simulink model "HevP2ReferenceApplication"  (R2022a)
settings: Solver=ode23tb  StartTime=0  StopTime=2474  RelTol=1e-2  EnableMultiTasking=on
undefined symbols (not defined in the file or in its folder): sigbuilder_block, SOCLast
libraries: simulink x5, autolibshared x2
(part 1 of 2)
settings Model: DataDictionary=HevP2ReferenceApplication.sldd  ModifiedByFormat=The MathWorks, Inc.  SimulationMode=accelerator  PauseTimes=23.46  Creator=The MathWorks, Inc.  LastModifiedBy=The MathWorks, Inc.
settings SolverCC: MaxConsecutiveMinStep=50  SolverJacobianMethodControl=FullPerturbation  ZeroCrossAlgorithm=Adaptive  AlgebraicLoopSolver=TrustRegion  AutoInsertRateTranBlk=on  DecoupledContinuousIntegration=on  MinimalZcImpactIntegration=on  MaxZcPerStep=1
settings DataIOCC: SaveOutput=off  DSMLogging=off  SaveTime=off  ReturnWorkspaceOutputs=off
settings OptimizationCC: EfficientMapNaN2IntZero=off
settings DebuggingCC: UnderspecifiedInitializationDetection=Classic  MergeDetectMultiDrivingBlocksExec=none  MaskedZcDiagnostic=none  IgnoredZcDiagnostic=none  UnconnectedInputMsg=warning  UnconnectedOutputMsg=warning  UnconnectedLineMsg=warning  ModelReferenceExtraNoncontSigs=none  PregeneratedLibrarySubsystemCodeDiagnostic=none  SFMachineParentedDataDiag=warning  ArithmeticOperatorsInVariantConditions=warning
settings HardwareCC: TargetBitPerLong=64  TargetBitPerPointer=64  TargetBitPerSizeT=64  TargetBitPerPtrDiffT=64  TargetLongLongMode=on  TargetIntDivRoundTo=Zero  TargetEndianess=LittleEndian  TargetWordSize=64  TargetHWDeviceType=MATLAB Host  ProdEqTarget=off
settings ModelReferenceCC: UpdateModelReferenceTargets=IfOutOfDate  ModelReferenceMinAlgLoopOccurrences=on  PropagateSignalLabelsOutOfModel=off
settings SFSimCC: SimUseLocalCustomCode=off
settings RTWCC: RTWUseLocalCustomCode=off  DLArmComputeVersion=19.05
settings CodeAppCC: MaxIdLength=128
settings GRTTargetCC: TargetLangStandard=C89/C90 (ANSI)  CombineOutputUpdateFcns=off  GRTInterface=on
settings ConfigComp: CovMetricSettings=dsw  CovSaveCumulativeToWorkspaceVar=on  CovSaveSingleToWorkspaceVar=on  CovExternalEMLEnable=off

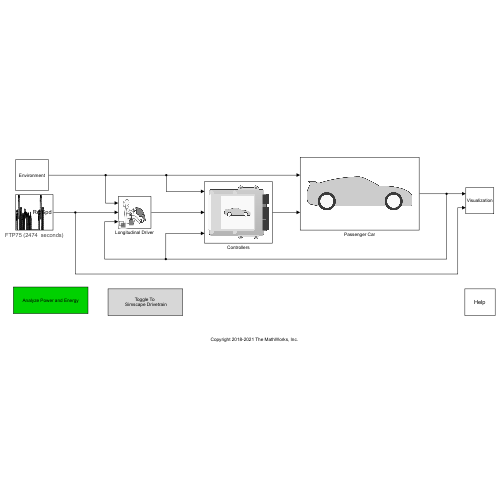
[thumbnail: Simulink's stored preview of the top-level diagram]
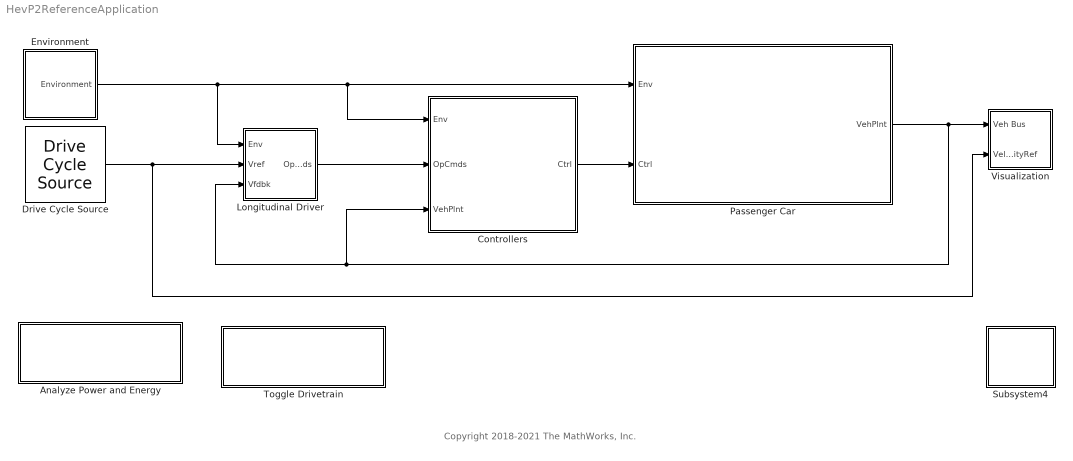
== system HevP2ReferenceApplication ==
  note: Copyright 2018-2021 The MathWorks, Inc.
  Analyze Power and Energy : Subsystem
      settings: OpenFcn=edit GenerateEnergyReport
      mask Display: disp(getString(message('autoblks:autoblkVehMask:powAndEne')))
  Controllers : Subsystem
      mask Display: image('SystemControllers.png', 'center')
  Drive Cycle Source : autolibshared/Drive Cycle Source  cycleVar=FTP75  fileVar=L:\Bauto\matlab\test\toolbox\shared\autoblks\scenario\adac.txt  tfinal="2474  seconds"  cycleRepeat=off  outAccPort=off  outGearPort=off  gearList=No gear data  t_wot1=1  xdot_woto=0  xdot_wot1=26.8  t_wot2=30  xdot_wot2=0  t_wotend=40  srcUnit=m/s  outUnit=m/s  srcAccUnit=m/s/s  outAccUnit=m/s^2  dt=0  aMode=1  faultOption=off  velBnd=2  velBndUnit=mph  inUnit=m/s  timeBnd=1  failOption=off  stopSim=off  maxFaultCnt=10  maxFaultTime=2  maxTotFaultTime=15  traceOption=off  dtTrace=1  traceWindow=10  lastDCname=FTP75  lastOutUnit=mph  lastDT=0  lastTB=1  lastSB=2  forceCalcBound=off
      settings: SourceProductBaseCode=PW,DR,MT,VE
  Environment : Subsystem
      mask Display: disp(getString(message('autoblks:autoblkVehMask:environ')))
  Longitudinal Driver : Subsystem  Variant=on  VariantControlMode=label  VariantControl=Variant1  LabelModeActiveChoice=0
      mask Display:
      | if strcmp('1',get_param(gcb,'ActiveVariant'))
      |     disp('Open Loop')
      | else
      |     image('LongitudinalDriver.png','center');
      | end
  Passenger Car : Subsystem
      mask Display: image('PassengerVehicle.png', 'center')
  Subsystem4 : Subsystem
      settings: OpenFcn=helpview([docroot,'/toolbox/autoblks/helptargets.map'], 'p2_hybrid_refapp')
      mask Display: disp(getString(message('autoblks:autoblkVehMask:help')))
  Toggle Drivetrain : Subsystem  mask(Drivetrain Model Selection){drivetrainMode=Powertrain Blockset}
      mask help: autoblks:autoblkHEVPx:ToggleDrivetrainSimscapeDesc
      settings: OpenFcn=open_system(gcb,'Mask')
      mask Help: eval('autosharedhelp(''p2_hybrid_refapp'')');
      mask TypeOptions drivetrainMode: Powertrain Blockset | Simscape
      mask Callback drivetrainMode:
      | if(strcmp(get_param(bdroot,'simulationstatus'),'stopped')) % only execute if simulation is stopped
      |     switch get_param(gcb,'drivetrainMode')
      |         case "Powertrain Blockset"
      |             set_param(bdroot,'Solver','ode23tb')
      |             set_param([bdroot '/Passenger Car/Drivetrain'], 'OverrideUsingVariant', 'Powertrain Blockset');
      |         case "Simscape"
      |             set_param(bdroot,'Solver','ode23t')
      |             set_param([bdroot '/Passenger Car/Drivetrain'], 'OverrideUsingVariant', 'Simscape');
      |         otherwise
      |             set_param(bdroot,'Solver','ode23tb')
      |             set_param([bdroot '/Passenger Car/Drivetrain'], 'OverrideUsingVariant', 'PTBS');
      |     end
      | end
      mask DialogControl ParameterGroupVar Prompt: Model Type
      mask Display:
      | if strcmp(get_param([bdroot(gcb) '/Passenger Car/Drivetrain'],'LabelModeActiveChoice'),'Powertrain Blockset')
      |    disp('Toggle To \n Simscape Drivetrain');
      | else
      |    disp('Toggle To \n Powertrain Blockset Drivetrain');
      | end
  Visualization : Subsystem
      mask Display: disp(getString(message('autoblks:autoblkVehMask:visual')))
  wires:
  Longitudinal Driver/1(" OpCmds") -> Controllers/2(OpCmds)
  Drive Cycle Source/1 -> Visualization/2(VelocityRef), Longitudinal Driver/2("Vref ")
  Environment/1(Environment) -> Passenger Car/1(Env), Controllers/1(Env), Longitudinal Driver/1(Env)
  Controllers/1(Ctrl) -> Passenger Car/2(Ctrl)
  Passenger Car/1(VehPlnt) -> Longitudinal Driver/3("Vfdbk "), Controllers/3(VehPlnt), Visualization/1(Veh Bus)

== system HevP2ReferenceApplication/Analyze Power and Energy ==

== system HevP2ReferenceApplication/Controllers ==
  Env : Inport
  OpCmds : Inport  Port=2
  VehPlnt : Inport  Port=3
  Bus Creator : BusCreator  Inputs=2
  PCM Input : Subsystem
  PCM Output : Subsystem
  Powertrain Control Module (PCM) : Subsystem
  Ctrl : Outport  VectorParamsAs1DForOutWhenUnconnected=off
  wires:
  Bus Creator/1 -> Ctrl/1
  [EngCtrl] -> Bus Creator/1
  [PtCtrl] -> Bus Creator/2
  Env/1 -> [Environment]
  VehPlnt/1 -> [VehPlnt]
  OpCmds/1 -> [OpCmds]
  PCM Input/27(BattSoc) -> Powertrain Control Module (PCM)/27(BattSoc)
  PCM Input/22(Ect) -> Powertrain Control Module (PCM)/22(Ect)
  PCM Input/23(EgrDeltaPrs) -> Powertrain Control Module (PCM)/23(EgrVlvDeltaPrs)
  PCM Input/5(ThrPosPct) -> Powertrain Control Module (PCM)/5(ThrPosPct)
  Powertrain Control Module (PCM)/7(ExhCamPhaseCmd) -> PCM Output/7(ExhCamPhaseCmd)
  PCM Input/32(EngTrqOut) -> Powertrain Control Module (PCM)/32(EngTrqOut)
  PCM Input/24(EgrInTemp) -> Powertrain Control Module (PCM)/24(EgrVlvInTemp)
  PCM Input/25(VehSpdFdbk) -> Powertrain Control Module (PCM)/25(VehSpdFdbk)
  PCM Input/12(IntkVlvLift) -> Powertrain Control Module (PCM)/12(IntkVlvLift)
  PCM Input/11(VarCompRatioPos) -> Powertrain Control Module (PCM)/11(VarCompRatioPos)
  PCM Input/26(EngSpdFdbk) -> Powertrain Control Module (PCM)/26(EngSpdFdbk)
  PCM Input/15(IntkSwirlVlvPos) -> Powertrain Control Module (PCM)/15(IntkSwirlVlvPos)
  Powertrain Control Module (PCM)/5(SpdAdv) -> PCM Output/5(SpkAdv)
  Powertrain Control Module (PCM)/13(ClsdLpFuelMult) -> PCM Output/13(ClsdLpFuelMult)
  PCM Input/28(BattPwr) -> Powertrain Control Module (PCM)/28(BattPwr)
  PCM Input/16(TurboSpd) -> Powertrain Control Module (PCM)/16(TurboSpd)
  PCM Input/10(EgrVlvAreaPct) -> Powertrain Control Module (PCM)/10(EgrVlvAreaPct)
  PCM Input/9(TurboRackPos) -> Powertrain Control Module (PCM)/9(TurboRackPos)
  PCM Input/14(Afr) -> Powertrain Control Module (PCM)/14(Afr)
  PCM Input/17(AmbPrs) -> Powertrain Control Module (PCM)/17(AmbPrs)
  PCM Input/13(VarIntkRunLen) -> Powertrain Control Module (PCM)/13(VarIntkRunLen)
  PCM Input/21(Iat) -> Powertrain Control Module (PCM)/21(Iat)
  Powertrain Control Module (PCM)/15(TrqCmdISC) -> PCM Output/15(TrqCmdISC)
  PCM Input/18(AccelPdl) -> Powertrain Control Module (PCM)/18(AccelPdl)
  Powertrain Control Module (PCM)/4(FuelMainSoi) -> PCM Output/4(FuelMainSoi)
  [Environment] -> PCM Input/2(Env)
  PCM Input/6(WgAreaPct) -> Powertrain Control Module (PCM)/6(WgAreaPct)
  Powertrain Control Module (PCM)/12(VarIntkRunLenCmd) -> PCM Output/12(VarIntkRunLenCmd)
  PCM Input/19(DecelPdl) -> Powertrain Control Module (PCM)/19(DecelPdl)
  PCM Input/1(TrqCmd) -> Powertrain Control Module (PCM)/1(TrqCmd)
  PCM Input/4(Mat) -> Powertrain Control Module (PCM)/4(Mat)
  Powertrain Control Module (PCM)/11(IntkVlvLiftCmd) -> PCM Output/11(IntkVlvLiftCmd)
  Powertrain Control Module (PCM)/18(EngTrqCmd) -> PCM Output/18(EngTrqCmd)
  PCM Input/3(Map) -> Powertrain Control Module (PCM)/3(Map)
  Powertrain Control Module (PCM)/21(BrkCmd) -> PCM Output/21(BrkCmd)
  PCM Input/20(IgnSwtch) -> Powertrain Control Module (PCM)/20(IgnSwtch)
  Powertrain Control Module (PCM)/16(LoadCmd) -> PCM Output/16(LoadCmd)
  PCM Input/7(IntkCamPhase) -> Powertrain Control Module (PCM)/7(IntkCamPhase)
  [PtCtrl] -> PCM Input/1(PtCtrl)
  Powertrain Control Module (PCM)/6(IntkCamPhaseCmd) -> PCM Output/6(IntkCamPhaseCmd)
  PCM Output/2(PtCtrl) -> [PtCtrl]
  Powertrain Control Module (PCM)/19(StartCmd) -> PCM Output/19(StartCmd)
  PCM Input/2(EngSpd) -> Powertrain Control Module (PCM)/2(EngSpd)
  Powertrain Control Module (PCM)/10(VarCompRatioPosCmd) -> PCM Output/10(VarCompRatioPosCmd)
  Powertrain Control Module (PCM)/17(EstIntkPortFlw) -> PCM Output/17(EstIntkPortFlw)
  [VehPlnt] -> PCM Input/3(VehPlnt)
  Powertrain Control Module (PCM)/9(EgrVlvAreaPctCmd) -> PCM Output/9(EgrVlvAreaPctCmd)
  Powertrain Control Module (PCM)/1(ThrPosPctCmd) -> PCM Output/1(ThrPosPctCmd)
  Powertrain Control Module (PCM)/2(WgAreaPctCmd) -> PCM Output/2(WgAreaPctCmd)
  [OpCmds] -> PCM Input/4(OpCmds)
  PCM Input/8(ExhCamPhase) -> Powertrain Control Module (PCM)/8(ExhCamPhase)
  Powertrain Control Module (PCM)/3(InjPw) -> PCM Output/3(InjPw)
  Powertrain Control Module (PCM)/14(IntkSwirlVlvPosCmd) -> PCM Output/14(IntkSwirlVlvPosCmd)
  PCM Input/29(MotSpd) -> Powertrain Control Module (PCM)/29(MotSpd)
  Powertrain Control Module (PCM)/8(TurboRackPosCmd) -> PCM Output/8(TurboRackPosCmd)
  PCM Output/1(EngCtrl) -> [EngCtrl]
  PCM Input/30(Cltch1State) -> Powertrain Control Module (PCM)/30(Cltch1State)
  PCM Input/31(Cltch2State) -> Powertrain Control Module (PCM)/31(Cltch2State)
  Powertrain Control Module (PCM)/22(GearCmd) -> PCM Output/22(GearCmd)
  Powertrain Control Module (PCM)/23(Cltch1Cmd) -> PCM Output/23(Cltch1Cmd)
  PCM Input/33(Chrg) -> Powertrain Control Module (PCM)/33(Chrg)
  Powertrain Control Module (PCM)/20(MotTrqCmd) -> PCM Output/20(MotTrqCmd)
  PCM Input/34(BattV) -> Powertrain Control Module (PCM)/34(BattV)
  PCM Input/35(TransGear) -> Powertrain Control Module (PCM)/35(TransGear)

== system HevP2ReferenceApplication/Environment ==
  Bus Creator : BusCreator  Inputs=4
  Bus Creator3 : BusCreator  Inputs=3
  Bus Creator4 : BusCreator  Inputs=2
  Bus Creator5 : BusCreator  Inputs=2
  Constant2 : Constant  Value=0
  Constant3 : Constant  Value=0
  Constant6 : Constant  Value=300
  Constant7 : Constant  Value=101325
  Ground{,1..3} (4 alike) : Ground
  Environment : Outport  VectorParamsAs1DForOutWhenUnconnected=off
  wires:
  Ground2/1 -> Bus Creator5/1  "lam_mu_x"
  Ground3/1 -> Bus Creator5/2  "lam_mu_y"
  Bus Creator5/1 -> Bus Creator4/2  "Ground_mu"
  Bus Creator4/1 -> Bus Creator/3  "Ground"
  Bus Creator3/1 -> Bus Creator/4  "Wind"
  Constant3/1 -> Bus Creator3/1  "wind_x"
  Ground/1 -> Bus Creator3/2  "wind_y"
  Ground1/1 -> Bus Creator3/3  "wind_z"
  Constant6/1 -> Bus Creator/1  "Temp"
  Constant2/1 -> Bus Creator4/1  "Grade"
  Bus Creator/1 -> Environment/1  "Environment"
  Constant7/1 -> Bus Creator/2  "Baro"

== system HevP2ReferenceApplication/Longitudinal Driver ==
  note: To switch variants, right-click on this subsystem (from one level above) and chose:
      | Variant, Active choice, <your selection>
  Env : Inport
  "Vref " : Inport  Port=2
  "Vfdbk " : Inport  Port=3
  Longitudinal Driver : Subsystem  VariantControl=0
      mask Display: image('LongitudinalDriver.png', 'center')
  Open Loop : Subsystem  VariantControl=1
      mask Display: disp('Open Loop')
  " OpCmds" : Outport  VectorParamsAs1DForOutWhenUnconnected=off

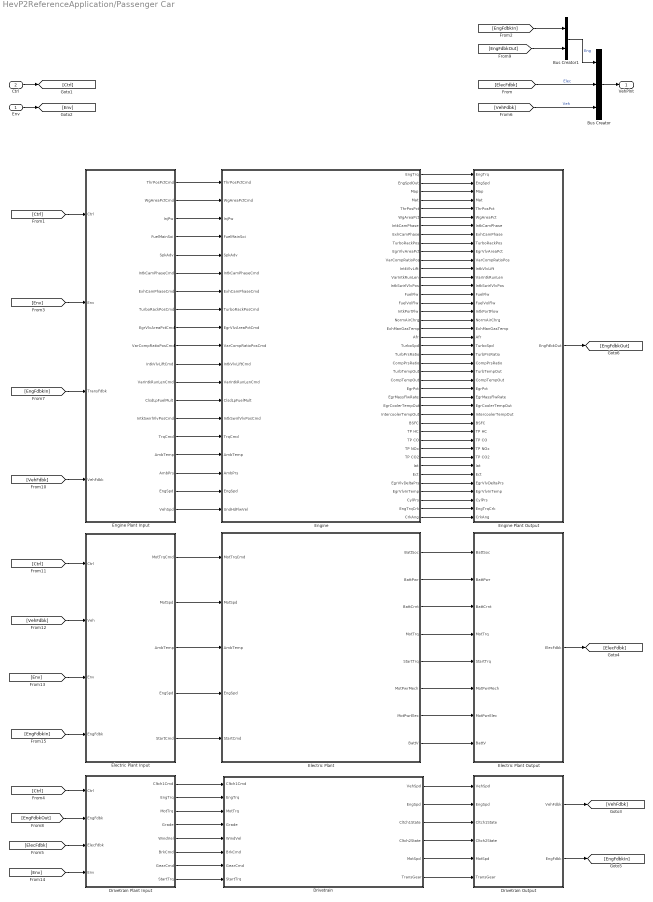
== system HevP2ReferenceApplication/Passenger Car ==
  Env : Inport
  Ctrl : Inport  Port=2
  Bus Creator : BusCreator  Inputs=3
  Bus Creator1 : BusCreator  Inputs=2
  Drivetrain : Subsystem  Variant=on  VariantControlMode=label  LabelModeActiveChoice=Powertrain Blockset
  Drivetrain Output : Subsystem
  Drivetrain Plant Input : Subsystem
  Electric Plant : Subsystem
  Electric Plant Input : Subsystem
  Electric Plant Output : Subsystem
  Engine : Subsystem  Variant=on  VariantControlMode=label  LabelModeActiveChoice=SiMappedEngine
  Engine Plant Input : Subsystem
  Engine Plant Output : Subsystem
  VehPlnt : Outport  VectorParamsAs1DForOutWhenUnconnected=off
  wires:
  [Ctrl] -> Drivetrain Plant Input/1(Ctrl)
  [EngFdbkOut] -> Drivetrain Plant Input/2(EngFdbk)
  Drivetrain/1(VehSpd) -> Drivetrain Output/1(VehSpd)
  Electric Plant Output/1(ElecFdbk) -> [ElecFdbk]
  [Ctrl] -> Electric Plant Input/1(Ctrl)
  [ElecFdbk] -> Drivetrain Plant Input/3(ElecFdbk)
  Drivetrain Plant Input/3(MotTrq) -> Drivetrain/3(MotTrq)
  Drivetrain Plant Input/1(Cltch1Cmd) -> Drivetrain/1(Cltch1Cmd)
  Drivetrain Plant Input/2(EngTrq) -> Drivetrain/2(EngTrq)
  [VehFdbk] -> Electric Plant Input/2(Veh)
  Electric Plant Input/1(MotTrqCmd) -> Electric Plant/1(MotTrqCmd)
  Electric Plant Input/2(MotSpd) -> Electric Plant/2(MotSpd)
  Electric Plant/1(BattSoc) -> Electric Plant Output/1(BattSoc)
  Electric Plant/2(BattPwr) -> Electric Plant Output/2(BattPwr)
  Electric Plant/3(BattCrnt) -> Electric Plant Output/3(BattCrnt)
  Electric Plant/4(MotTrq) -> Electric Plant Output/4(MotTrq)
  [Env] -> Electric Plant Input/3(Env)
  Electric Plant Input/3(AmbTemp) -> Electric Plant/3(AmbTemp)
  [Env] -> Drivetrain Plant Input/4(Env)
  Drivetrain Plant Input/4(Grade) -> Drivetrain/4(Grade)
  Drivetrain Plant Input/5(WindVel) -> Drivetrain/5(WindVel)
  [EngFdbkIn] -> Electric Plant Input/4(EngFdbk)
  Electric Plant Input/4(EngSpd) -> Electric Plant/4(EngSpd)
  Electric Plant/5(StartTrq) -> Electric Plant Output/5(StartTrq)
  Electric Plant Input/5(StartCmd) -> Electric Plant/5(StartCmd)
  Engine Plant Input/17(AmbPrs) -> Engine/17(AmbPrs)
  [EngFdbkIn] -> Bus Creator1/1
  Engine Plant Input/6(IntkCamPhaseCmd) -> Engine/6(IntkCamPhaseCmd)
  Engine Plant Input/12(VarIntkRunLenCmd) -> Engine/12(VarIntkRunLenCmd)
  [EngFdbkIn] -> Engine Plant Input/3(TransFdbk)
  Engine Plant Input/16(AmbTemp) -> Engine/16(AmbTemp)
  Bus Creator/1 -> VehPlnt/1
  Engine Plant Input/14(IntkSwirlVlvPosCmd) -> Engine/14(IntkSwirlVlvPosCmd)
  [ElecFdbk] -> Bus Creator/2  "Elec"
  Engine Plant Input/5(SpkAdv) -> Engine/5(SpkAdv)
  Engine Plant Output/1(EngFdbkOut) -> [EngFdbkOut]
  Env/1 -> [Env]
  [EngFdbkOut] -> Bus Creator1/2
  Engine Plant Input/7(ExhCamPhaseCmd) -> Engine/7(ExhCamPhaseCmd)
  Engine Plant Input/1(ThrPosPctCmd) -> Engine/1(ThrPosPctCmd)
  Engine Plant Input/19(VehSpd) -> Engine/19(UndHdFlwVel)
  Engine Plant Input/9(EgrVlvAreaPctCmd) -> Engine/9(EgrVlvAreaPctCmd)
  [Env] -> Engine Plant Input/2(Env)
  Engine Plant Input/3(InjPw) -> Engine/3(InjPw)
  Engine Plant Input/11(IntkVlvLiftCmd) -> Engine/11(IntkVlvLiftCmd)
  [VehFdbk] -> Engine Plant Input/4(VehFdbk)
  Engine Plant Input/4(FuelMainSoi) -> Engine/4(FuelMainSoi)
  Engine Plant Input/18(EngSpd) -> Engine/18(EngSpd)
  Engine Plant Input/8(TurboRackPosCmd) -> Engine/8(TurboRackPosCmd)
  Engine Plant Input/2(WgAreaPctCmd) -> Engine/2(WgAreaPctCmd)
  [Ctrl] -> Engine Plant Input/1(Ctrl)
  Engine Plant Input/13(ClsdLpFuelMult) -> Engine/13(ClsdLpFuelMult)
  Engine Plant Input/10(VarCompRatioPosCmd) -> Engine/10(VarCompRatioPosCmd)
  Bus Creator1/1 -> Bus Creator/1  "Eng"
  Ctrl/1 -> [Ctrl]
  Engine Plant Input/15(TrqCmd) -> Engine/15(TrqCmd)
  [VehFdbk] -> Bus Creator/3  "Veh"
  Electric Plant/6(MotPwrMech) -> Electric Plant Output/6(MotPwrMech)
  Electric Plant/7(MotPwrElec) -> Electric Plant Output/7(MotPwrElec)
  Electric Plant/8(BattV) -> Electric Plant Output/8(BattV)
  Engine/1(EngTrq) -> Engine Plant Output/1(EngTrq)
  Engine/2(EngSpdOut) -> Engine Plant Output/2(EngSpd)
  Engine/3(Map) -> Engine Plant Output/3(Map)
  Engine/4(Mat) -> Engine Plant Output/4(Mat)
  Engine/5(ThrPosPct) -> Engine Plant Output/5(ThrPosPct)
  Engine/6(WgAreaPct) -> Engine Plant Output/6(WgAreaPct)
  Engine/7(IntkCamPhase) -> Engine Plant Output/7(IntkCamPhase)
  Engine/8(ExhCamPhase) -> Engine Plant Output/8(ExhCamPhase)
  Engine/9(TurboRackPos) -> Engine Plant Output/9(TurboRackPos)
  Engine/10(EgrVlvAreaPct) -> Engine Plant Output/10(EgrVlvAreaPct)
  Engine/11(VarCompRatioPos) -> Engine Plant Output/11(VarCompRatioPos)
  Engine/12(IntkVlvLift) -> Engine Plant Output/12(IntkVlvLift)
  Engine/13(VarIntkRunLen) -> Engine Plant Output/13(VarIntkRunLen)
  Engine/14(IntkSwirlVlvPos) -> Engine Plant Output/14(IntkSwirlVlvPos)
  Engine/15(FuelFlw) -> Engine Plant Output/15(FuelFlw)
  Engine/16(FuelVolFlw) -> Engine Plant Output/16(FuelVolFlw)
  Engine/17(IntkPortFlw) -> Engine Plant Output/17(IntkPortFlow)
  Engine/18(NormAirChrg) -> Engine Plant Output/18(NormAirChrg)
  Engine/19(ExhManGasTemp) -> Engine Plant Output/19(ExhManGasTemp)
  Engine/20(Afr) -> Engine Plant Output/20(Afr)
  Engine/21(TurboSpd) -> Engine Plant Output/21(TurboSpd)
  Engine/22(TurbPrsRatio) -> Engine Plant Output/22(TurbPrsRatio)
  Engine/23(CompPrsRatio) -> Engine Plant Output/23(CompPrsRatio)
  Engine/24(TurbTempOut) -> Engine Plant Output/24(TurbTempOut)
  Engine/25(CompTempOut) -> Engine Plant Output/25(CompTempOut)
  Engine/26(EgrPct) -> Engine Plant Output/26(EgrPct)
  Engine/27(EgrMassFlwRate) -> Engine Plant Output/27(EgrMassFlwRate)
  Engine/28(EgrCoolerTempOut) -> Engine Plant Output/28(EgrCoolerTempOut)
  Engine/29(IntercoolerTempOut) -> Engine Plant Output/29(IntercoolerTempOut)
  Engine/30(BSFC) -> Engine Plant Output/30(BSFC)
  Engine/31(TP HC) -> Engine Plant Output/31(TP HC)
  Engine/32(TP CO) -> Engine Plant Output/32(TP CO)
  Engine/33(TP NOx) -> Engine Plant Output/33(TP NOx)
  Engine/34(TP CO2) -> Engine Plant Output/34(TP CO2)
  Engine/35(Iat) -> Engine Plant Output/35(Iat)
  Engine/36(Ect) -> Engine Plant Output/36(Ect)
  Engine/37(EgrVlvDeltaPrs) -> Engine Plant Output/37(EgrVlvDeltaPrs)
  Engine/38(EgrVlvInTemp) -> Engine Plant Output/38(EgrVlvInTemp)
  Engine/39(CylPrs) -> Engine Plant Output/39(CylPrs)
  Engine/40(EngTrqCrk) -> Engine Plant Output/40(EngTrqCrk)
  Engine/41(CrkAng) -> Engine Plant Output/41(CrkAng)
  Drivetrain/4(Cltch2State) -> Drivetrain Output/4(Cltch2State)
  Drivetrain/3(Cltch1State) -> Drivetrain Output/3(Cltch1State)
  Drivetrain Output/2(EngFdbk) -> [EngFdbkIn]
  Drivetrain Output/1(VehFdbk) -> [VehFdbk]
  Drivetrain/6(TransGear) -> Drivetrain Output/6(TransGear)
  Drivetrain/2(EngSpd) -> Drivetrain Output/2("EngSpd ")
  Drivetrain/5(MotSpd) -> Drivetrain Output/5(MotSpd)
  Drivetrain Plant Input/7(GearCmd) -> Drivetrain/7(GearCmd)
  Drivetrain Plant Input/8(StartTrq) -> Drivetrain/8(StartTrq)
  Drivetrain Plant Input/6(BrkCmd) -> Drivetrain/6(BrkCmd)

== system HevP2ReferenceApplication/Subsystem4 ==

== system HevP2ReferenceApplication/Toggle Drivetrain ==

== system HevP2ReferenceApplication/Visualization ==
  Veh Bus : Inport
  VelocityRef : Inport  Port=2
  Bus Selector1 : BusSelector  OutputSignals=Veh.xdot,Eng.EngFdbkOut.EngSpd,Veh.MotSpd,Eng.EngFdbkOut.EngTrq,Elec.MotTrq,Elec.BattCrnt,Elec.BattSoc,Eng.EngFdbkOut.Afr,Eng.EngFdbkOut.FuelVolFlw,Elec.BattPwr,Eng.EngFdbkOut.TP HC,Eng.EngFdbkOut.TP CO,Eng.EngFdbkOut.TP NOx,Eng.EngFdbkOut.TP CO2
  Emission Calculations : Subsystem
  Mux : Mux  Inputs=2
  Mux1 : Mux  Inputs=2
  Mux2 : Mux  Inputs=2
  Performance Calculations : Subsystem
  Performance and FE Scope : Scope  NumInputPorts=6
  Rate Transition{1..2,4..5,7..8,10} (7 alike) : RateTransition  Deterministic=off
  TP Emissions Scope : Scope  NumInputPorts=4
  Terminator : Terminator
  Terminator1 : Terminator
  m/s to mph : Gain  Gain=2.23694
  rad/s to rpm : Gain  Gain=30/pi
  wires:
  Veh Bus/1 -> Bus Selector1/1
  Bus Selector1/1 -> Performance Calculations/1(VehSpd), Mux/2  "<xdot>"
  Bus Selector1/2 -> Rate Transition2/1  "<EngSpd>"
  Mux/1 -> m/s to mph/1
  Bus Selector1/9 -> Performance Calculations/2(FuelVolFlow)  "<FuelVolFlw>"
  Performance Calculations/1(US MPG) -> Performance and FE Scope/6  "US Fuel Economy MPGe"
  Performance Calculations/2(L/100Km) -> Terminator/1
  Bus Selector1/8 -> Terminator1/1  "<Afr>"
  m/s to mph/1 -> Rate Transition4/1
  Bus Selector1/7 -> Rate Transition1/1  "<BattSoc>"
  Bus Selector1/11 -> Emission Calculations/2(TP HC Mass Flow)  "<TP HC>"
  Bus Selector1/12 -> Emission Calculations/3(TP CO Mass Flow)  "<TP CO>"
  Bus Selector1/13 -> Emission Calculations/4(TP NOx Mass Flow)  "<TP NOx>"
  Emission Calculations/1(TP HC Mass) -> TP Emissions Scope/1
  Emission Calculations/2(TP CO Mass) -> TP Emissions Scope/2
  Emission Calculations/3(TP NOx Mass) -> TP Emissions Scope/3
  Bus Selector1/14 -> Emission Calculations/5(TP CO2 Mass Flow)  "<TP CO2>"
  Emission Calculations/4(TP CO2 Mass) -> TP Emissions Scope/4
  VelocityRef/1 -> Emission Calculations/1(VehSpd), Mux/1
  Rate Transition1/1 -> Performance and FE Scope/5  "Battery SOC"
  Mux1/1 -> Performance and FE Scope/2  "EngSpd, MotSpd (RPM)"
  Rate Transition4/1 -> Performance and FE Scope/1  "Trace Velocity, Target, Actual (mph)"
  Bus Selector1/10 -> Performance Calculations/3(BattPwr)  "<BattPwr>"
  Bus Selector1/3 -> rad/s to rpm/1  "<MotSpd>"
  Rate Transition2/1 -> Mux1/1
  Rate Transition5/1 -> Mux1/2
  Rate Transition8/1 -> Mux2/2
  Rate Transition7/1 -> Mux2/1
  Mux2/1 -> Performance and FE Scope/3  "EngTrq, MotTrq (Nm)"
  Bus Selector1/4 -> Rate Transition7/1  "<EngTrq>"
  Bus Selector1/5 -> Rate Transition8/1  "<MotTrq>"
  Bus Selector1/6 -> Rate Transition10/1  "<BattCrnt>"
  Rate Transition10/1 -> Performance and FE Scope/4  "Battery Current (A)"
  rad/s to rpm/1 -> Rate Transition5/1

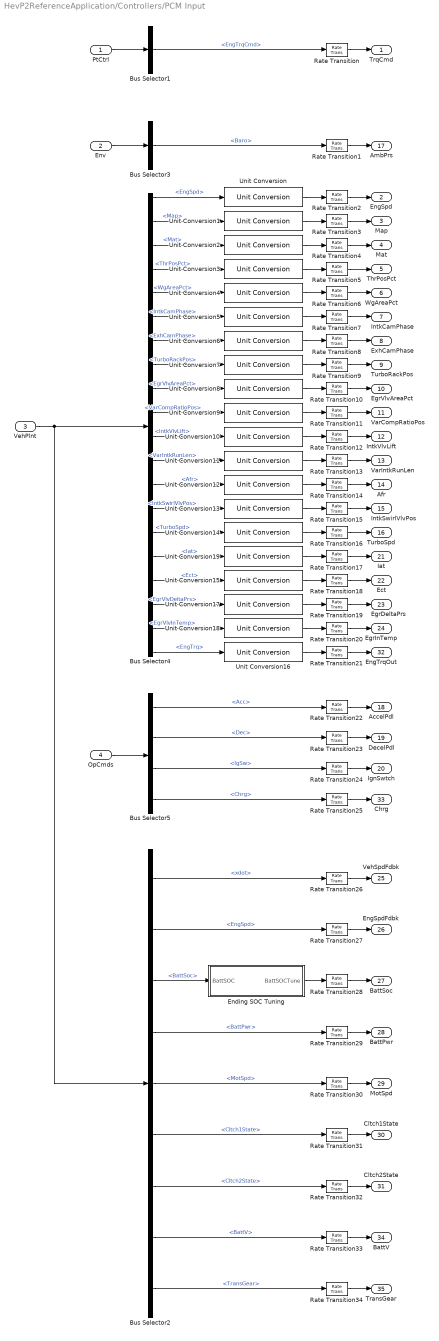
== system HevP2ReferenceApplication/Controllers/PCM Input ==
  PtCtrl : Inport
  Env : Inport  Port=2
  VehPlnt : Inport  Port=3
  OpCmds : Inport  Port=4
  Bus Selector1 : BusSelector  OutputSignals=EngTrqCmd
  Bus Selector2 : BusSelector  OutputSignals=Veh.xdot,Eng.EngFdbk.EngSpd,Elec.BattSoc,Elec.BattPwr,Veh.MotSpd,Veh.Cltch1State,Veh.Cltch2State,Elec.BattV,Veh.TransGear
  Bus Selector3 : BusSelector  OutputSignals=Baro
  Bus Selector4 : BusSelector  OutputSignals=Eng.EngFdbkOut.EngSpd,Eng.EngFdbkOut.Map,Eng.EngFdbkOut.Mat,Eng.EngFdbkOut.ThrPosPct,Eng.EngFdbkOut.WgAreaPct,Eng.EngFdbkOut.IntkCamPhase,Eng.EngFdbkOut.ExhCamPhase,Eng.EngFdbkOut.TurboRackPos,Eng.EngFdbkOut.EgrVlvAreaPct,Eng.EngFdbkOut.VarCompRatioPos,Eng.EngFdbkOut.IntkVlvLift,Eng.EngFdbkOut.VarIntkRunLen,Eng.EngFdbkOut.Afr,Eng.EngFdbkOut.IntkSwirlVlvPos,Eng.EngFdbkOut.TurboSpd,Eng.EngFdbkOut.Iat,Eng.EngFdbkOut.Ect,Eng.EngFdbkOut.EgrVlvDeltaPrs,Eng.EngFdbkOut.EgrVlvInTemp,Eng.EngFdbkOut.EngTrq
  Bus Selector5 : BusSelector  OutputSignals=Acc,Dec,IgSw,Chrg
  Ending SOC Tuning : Subsystem  Variant=on  VariantControlMode=label  LabelModeActiveChoice=0
  Rate Transition{,1..34} (35 alike) : RateTransition
  Unit Conversion{,1..19} (20 alike) : UnitConversion
  TrqCmd : Outport  VectorParamsAs1DForOutWhenUnconnected=off
  EngSpd : Outport  Port=2  VectorParamsAs1DForOutWhenUnconnected=off
  Map : Outport  Port=3  VectorParamsAs1DForOutWhenUnconnected=off
  Mat : Outport  Port=4  VectorParamsAs1DForOutWhenUnconnected=off
  ThrPosPct : Outport  Port=5  VectorParamsAs1DForOutWhenUnconnected=off
  WgAreaPct : Outport  Port=6  VectorParamsAs1DForOutWhenUnconnected=off
  IntkCamPhase : Outport  Port=7  VectorParamsAs1DForOutWhenUnconnected=off
  ExhCamPhase : Outport  Port=8  VectorParamsAs1DForOutWhenUnconnected=off
  TurboRackPos : Outport  Port=9  VectorParamsAs1DForOutWhenUnconnected=off
  EgrVlvAreaPct : Outport  Port=10  VectorParamsAs1DForOutWhenUnconnected=off
  VarCompRatioPos : Outport  Port=11  VectorParamsAs1DForOutWhenUnconnected=off
  IntkVlvLift : Outport  Port=12  VectorParamsAs1DForOutWhenUnconnected=off
  VarIntkRunLen : Outport  Port=13  VectorParamsAs1DForOutWhenUnconnected=off
  Afr : Outport  Port=14  VectorParamsAs1DForOutWhenUnconnected=off
  IntkSwirlVlvPos : Outport  Port=15  VectorParamsAs1DForOutWhenUnconnected=off
  TurboSpd : Outport  Port=16  VectorParamsAs1DForOutWhenUnconnected=off
  AmbPrs : Outport  Port=17  VectorParamsAs1DForOutWhenUnconnected=off
  AccelPdl : Outport  Port=18  VectorParamsAs1DForOutWhenUnconnected=off
  DecelPdl : Outport  Port=19  VectorParamsAs1DForOutWhenUnconnected=off
  IgnSwtch : Outport  Port=20  VectorParamsAs1DForOutWhenUnconnected=off
  Iat : Outport  Port=21  VectorParamsAs1DForOutWhenUnconnected=off
  Ect : Outport  Port=22  VectorParamsAs1DForOutWhenUnconnected=off
  EgrDeltaPrs : Outport  Port=23  VectorParamsAs1DForOutWhenUnconnected=off
  EgrInTemp : Outport  Port=24  VectorParamsAs1DForOutWhenUnconnected=off
  VehSpdFdbk : Outport  Port=25  VectorParamsAs1DForOutWhenUnconnected=off
  EngSpdFdbk : Outport  Port=26  VectorParamsAs1DForOutWhenUnconnected=off
  BattSoc : Outport  Port=27  VectorParamsAs1DForOutWhenUnconnected=off
  BattPwr : Outport  Port=28  VectorParamsAs1DForOutWhenUnconnected=off
  MotSpd : Outport  Port=29  VectorParamsAs1DForOutWhenUnconnected=off
  Cltch1State : Outport  Port=30  VectorParamsAs1DForOutWhenUnconnected=off
  Cltch2State : Outport  Port=31  VectorParamsAs1DForOutWhenUnconnected=off
  EngTrqOut : Outport  Port=32  Unit=N*m  VectorParamsAs1DForOutWhenUnconnected=off
  Chrg : Outport  Port=33  VectorParamsAs1DForOutWhenUnconnected=off
  BattV : Outport  Port=34  VectorParamsAs1DForOutWhenUnconnected=off
  TransGear : Outport  Port=35  VectorParamsAs1DForOutWhenUnconnected=off
  wires:
  PtCtrl/1 -> Bus Selector1/1
  OpCmds/1 -> Bus Selector5/1
  VehPlnt/1 -> Bus Selector4/1, Bus Selector2/1
  Unit Conversion6/1 -> Rate Transition8/1
  Unit Conversion1/1 -> Rate Transition3/1
  Unit Conversion14/1 -> Rate Transition16/1
  Unit Conversion12/1 -> Rate Transition14/1
  Unit Conversion2/1 -> Rate Transition4/1
  Unit Conversion13/1 -> Rate Transition15/1
  Unit Conversion7/1 -> Rate Transition9/1
  Unit Conversion4/1 -> Rate Transition6/1
  Unit Conversion3/1 -> Rate Transition5/1
  Unit Conversion5/1 -> Rate Transition7/1
  Unit Conversion10/1 -> Rate Transition12/1
  Unit Conversion11/1 -> Rate Transition13/1
  Unit Conversion/1 -> Rate Transition2/1
  Unit Conversion9/1 -> Rate Transition11/1
  Unit Conversion8/1 -> Rate Transition10/1
  Unit Conversion15/1 -> Rate Transition18/1
  Unit Conversion16/1 -> Rate Transition21/1
  Env/1 -> Bus Selector3/1
  Unit Conversion17/1 -> Rate Transition19/1
  Unit Conversion18/1 -> Rate Transition20/1
  Unit Conversion19/1 -> Rate Transition17/1
  Bus Selector2/1 -> Rate Transition26/1  "<xdot>"
  Bus Selector2/2 -> Rate Transition27/1  "<EngSpd>"
  Bus Selector2/3 -> Ending SOC Tuning/1(BattSOC)  "<BattSoc>"
  Bus Selector2/4 -> Rate Transition29/1  "<BattPwr>"
  Bus Selector2/5 -> Rate Transition30/1  "<MotSpd>"
  Bus Selector2/6 -> Rate Transition31/1  "<Cltch1State>"
  Bus Selector2/7 -> Rate Transition32/1  "<Cltch2State>"
  Bus Selector2/8 -> Rate Transition33/1  "<BattV>"
  Bus Selector2/9 -> Rate Transition34/1  "<TransGear>"
  Bus Selector5/1 -> Rate Transition22/1  "<Acc>"
  Bus Selector5/2 -> Rate Transition23/1  "<Dec>"
  Bus Selector5/3 -> Rate Transition24/1  "<IgSw>"
  Bus Selector5/4 -> Rate Transition25/1  "<Chrg>"
  Bus Selector4/1 -> Unit Conversion/1  "<EngSpd>"
  Bus Selector4/2 -> Unit Conversion1/1  "<Map>"
  Bus Selector4/3 -> Unit Conversion2/1  "<Mat>"
  Bus Selector4/4 -> Unit Conversion3/1  "<ThrPosPct>"
  Bus Selector4/5 -> Unit Conversion4/1  "<WgAreaPct>"
  Bus Selector4/6 -> Unit Conversion5/1  "<IntkCamPhase>"
  Bus Selector4/7 -> Unit Conversion6/1  "<ExhCamPhase>"
  Bus Selector4/8 -> Unit Conversion7/1  "<TurboRackPos>"
  Bus Selector4/9 -> Unit Conversion8/1  "<EgrVlvAreaPct>"
  Bus Selector4/10 -> Unit Conversion9/1  "<VarCompRatioPos>"
  Bus Selector4/11 -> Unit Conversion10/1  "<IntkVlvLift>"
  Bus Selector4/12 -> Unit Conversion11/1  "<VarIntkRunLen>"
  Bus Selector4/13 -> Unit Conversion12/1  "<Afr>"
  Bus Selector4/14 -> Unit Conversion13/1  "<IntkSwirlVlvPos>"
  Bus Selector4/15 -> Unit Conversion14/1  "<TurboSpd>"
  Bus Selector4/16 -> Unit Conversion19/1  "<Iat>"
  Bus Selector4/17 -> Unit Conversion15/1  "<Ect>"
  Bus Selector4/18 -> Unit Conversion17/1  "<EgrVlvDeltaPrs>"
  Bus Selector4/19 -> Unit Conversion18/1  "<EgrVlvInTemp>"
  Bus Selector4/20 -> Unit Conversion16/1  "<EngTrq>"
  Bus Selector3/1 -> Rate Transition1/1  "<Baro>"
  Bus Selector1/1 -> Rate Transition/1  "<EngTrqCmd>"
  Rate Transition19/1 -> EgrDeltaPrs/1
  Rate Transition18/1 -> Ect/1
  Rate Transition2/1 -> EngSpd/1
  Rate Transition17/1 -> Iat/1
  Rate Transition6/1 -> WgAreaPct/1
  Rate Transition7/1 -> IntkCamPhase/1
  Rate Transition8/1 -> ExhCamPhase/1
  Rate Transition9/1 -> TurboRackPos/1
  Rate Transition4/1 -> Mat/1
  Rate Transition5/1 -> ThrPosPct/1
  Rate Transition11/1 -> VarCompRatioPos/1
  Rate Transition15/1 -> IntkSwirlVlvPos/1
  Rate Transition1/1 -> AmbPrs/1
  Rate Transition10/1 -> EgrVlvAreaPct/1
  Rate Transition13/1 -> VarIntkRunLen/1
  Rate Transition14/1 -> Afr/1
  Rate Transition3/1 -> Map/1
  Rate Transition20/1 -> EgrInTemp/1
  Rate Transition/1 -> TrqCmd/1
  Rate Transition12/1 -> IntkVlvLift/1
  Rate Transition16/1 -> TurboSpd/1
  Rate Transition21/1 -> EngTrqOut/1
  Rate Transition22/1 -> AccelPdl/1
  Rate Transition23/1 -> DecelPdl/1
  Rate Transition24/1 -> IgnSwtch/1
  Rate Transition25/1 -> Chrg/1
  Rate Transition26/1 -> VehSpdFdbk/1
  Rate Transition27/1 -> EngSpdFdbk/1
  Rate Transition28/1 -> BattSoc/1
  Rate Transition31/1 -> Cltch1State/1
  Rate Transition30/1 -> MotSpd/1
  Rate Transition29/1 -> BattPwr/1
  Rate Transition32/1 -> Cltch2State/1
  Rate Transition34/1 -> TransGear/1
  Rate Transition33/1 -> BattV/1
  Ending SOC Tuning/1(BattSOCTune) -> Rate Transition28/1

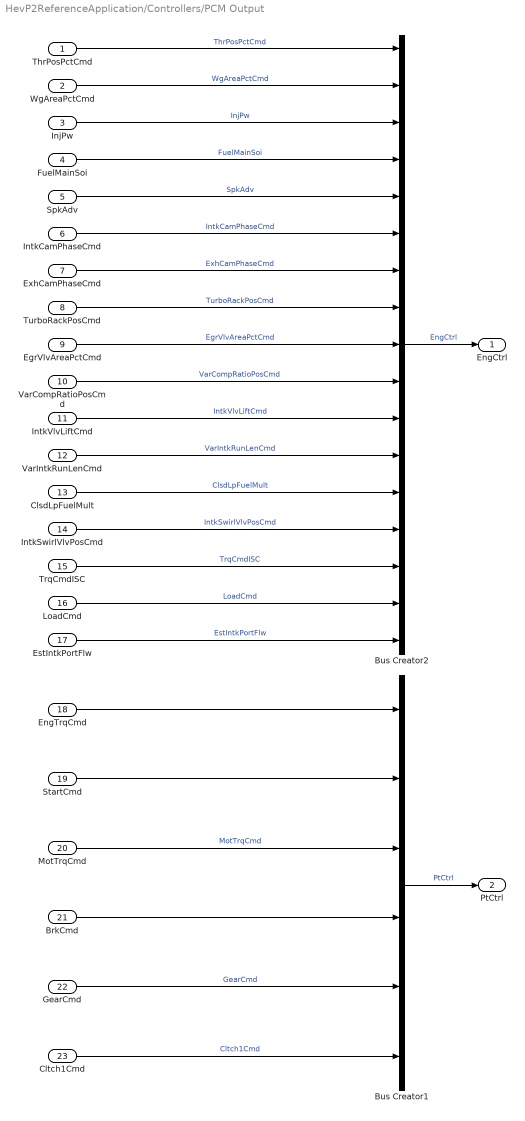
== system HevP2ReferenceApplication/Controllers/PCM Output ==
  ThrPosPctCmd : Inport
  WgAreaPctCmd : Inport  Port=2
  InjPw : Inport  Port=3
  FuelMainSoi : Inport  Port=4
  SpkAdv : Inport  Port=5
  IntkCamPhaseCmd : Inport  Port=6
  ExhCamPhaseCmd : Inport  Port=7
  TurboRackPosCmd : Inport  Port=8
  EgrVlvAreaPctCmd : Inport  Port=9
  VarCompRatioPosCmd : Inport  Port=10
  IntkVlvLiftCmd : Inport  Port=11
  VarIntkRunLenCmd : Inport  Port=12
  ClsdLpFuelMult : Inport  Port=13
  IntkSwirlVlvPosCmd : Inport  Port=14
  TrqCmdISC : Inport  Port=15
  LoadCmd : Inport  Port=16
  EstIntkPortFlw : Inport  Port=17
  EngTrqCmd : Inport  Port=18
  StartCmd : Inport  Port=19
  MotTrqCmd : Inport  Port=20
  BrkCmd : Inport  Port=21
  GearCmd : Inport  Port=22
  Cltch1Cmd : Inport  Port=23
  Bus Creator1 : BusCreator  Inputs=6
  Bus Creator2 : BusCreator  Inputs=17
  EngCtrl : Outport  VectorParamsAs1DForOutWhenUnconnected=off
  PtCtrl : Outport  Port=2  VectorParamsAs1DForOutWhenUnconnected=off
  wires:
  BrkCmd/1 -> Bus Creator1/4
  Bus Creator1/1 -> PtCtrl/1  "PtCtrl"
  EngTrqCmd/1 -> Bus Creator1/1
  StartCmd/1 -> Bus Creator1/2
  Bus Creator2/1 -> EngCtrl/1  "EngCtrl"
  LoadCmd/1 -> Bus Creator2/16  "LoadCmd"
  TurboRackPosCmd/1 -> Bus Creator2/8  "TurboRackPosCmd"
  InjPw/1 -> Bus Creator2/3  "InjPw"
  IntkSwirlVlvPosCmd/1 -> Bus Creator2/14  "IntkSwirlVlvPosCmd"
  FuelMainSoi/1 -> Bus Creator2/4  "FuelMainSoi"
  ThrPosPctCmd/1 -> Bus Creator2/1  "ThrPosPctCmd"
  VarIntkRunLenCmd/1 -> Bus Creator2/12  "VarIntkRunLenCmd"
  TrqCmdISC/1 -> Bus Creator2/15  "TrqCmdISC"
  IntkCamPhaseCmd/1 -> Bus Creator2/6  "IntkCamPhaseCmd"
  EgrVlvAreaPctCmd/1 -> Bus Creator2/9  "EgrVlvAreaPctCmd"
  WgAreaPctCmd/1 -> Bus Creator2/2  "WgAreaPctCmd"
  SpkAdv/1 -> Bus Creator2/5  "SpkAdv"
  EstIntkPortFlw/1 -> Bus Creator2/17  "EstIntkPortFlw"
  ClsdLpFuelMult/1 -> Bus Creator2/13  "ClsdLpFuelMult"
  VarCompRatioPosCmd/1 -> Bus Creator2/10  "VarCompRatioPosCmd"
  ExhCamPhaseCmd/1 -> Bus Creator2/7  "ExhCamPhaseCmd"
  IntkVlvLiftCmd/1 -> Bus Creator2/11  "IntkVlvLiftCmd"
  Cltch1Cmd/1 -> Bus Creator1/6  "Cltch1Cmd"
  GearCmd/1 -> Bus Creator1/5  "GearCmd"
  MotTrqCmd/1 -> Bus Creator1/3  "MotTrqCmd"

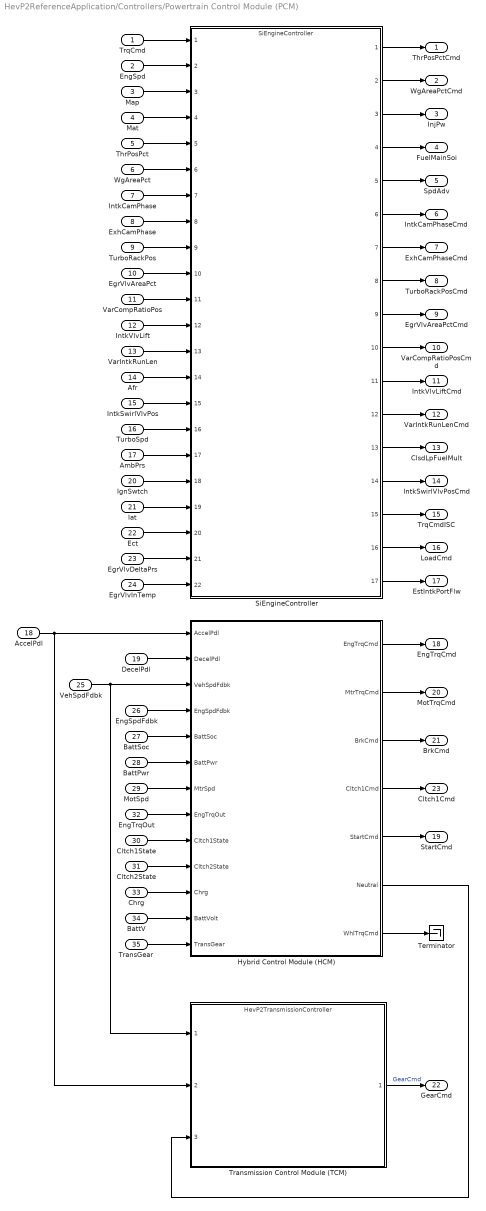
== system HevP2ReferenceApplication/Controllers/Powertrain Control Module (PCM) ==
  TrqCmd : Inport
  EngSpd : Inport  Port=2
  Map : Inport  Port=3
  Mat : Inport  Port=4
  ThrPosPct : Inport  Port=5
  WgAreaPct : Inport  Port=6
  IntkCamPhase : Inport  Port=7
  ExhCamPhase : Inport  Port=8
  TurboRackPos : Inport  Port=9
  EgrVlvAreaPct : Inport  Port=10
  VarCompRatioPos : Inport  Port=11
  IntkVlvLift : Inport  Port=12
  VarIntkRunLen : Inport  Port=13
  Afr : Inport  Port=14
  IntkSwirlVlvPos : Inport  Port=15
  TurboSpd : Inport  Port=16
  AmbPrs : Inport  Port=17
  AccelPdl : Inport  Port=18
  DecelPdl : Inport  Port=19
  IgnSwtch : Inport  Port=20
  Iat : Inport  Port=21
  Ect : Inport  Port=22
  EgrVlvDeltaPrs : Inport  Port=23
  EgrVlvInTemp : Inport  Port=24
  VehSpdFdbk : Inport  Port=25
  EngSpdFdbk : Inport  Port=26
  BattSoc : Inport  Port=27
  BattPwr : Inport  Port=28
  MotSpd : Inport  Port=29
  Cltch1State : Inport  Port=30
  Cltch2State : Inport  Port=31
  EngTrqOut : Inport  Port=32
  Chrg : Inport  Port=33
  BattV : Inport  Port=34
  TransGear : Inport  Port=35
  Hybrid Control Module (HCM) : Subsystem  Variant=on  VariantControlMode=label  LabelModeActiveChoice=OptimalControl
  SiEngineController : ModelReference  ModelNameDialog=SiEngineController.slx  SimulationMode=Normal  ModelReferenceVersion=4.6
  Terminator : Terminator
  Transmission Control Module (TCM) : ModelReference  ModelNameDialog=HevP2TransmissionController.slx  SimulationMode=Normal  ModelReferenceVersion=8.1
  ThrPosPctCmd : Outport  VectorParamsAs1DForOutWhenUnconnected=off
  WgAreaPctCmd : Outport  Port=2  VectorParamsAs1DForOutWhenUnconnected=off
  InjPw : Outport  Port=3  VectorParamsAs1DForOutWhenUnconnected=off
  FuelMainSoi : Outport  Port=4  VectorParamsAs1DForOutWhenUnconnected=off
  SpdAdv : Outport  Port=5  VectorParamsAs1DForOutWhenUnconnected=off
  IntkCamPhaseCmd : Outport  Port=6  VectorParamsAs1DForOutWhenUnconnected=off
  ExhCamPhaseCmd : Outport  Port=7  VectorParamsAs1DForOutWhenUnconnected=off
  TurboRackPosCmd : Outport  Port=8  VectorParamsAs1DForOutWhenUnconnected=off
  EgrVlvAreaPctCmd : Outport  Port=9  VectorParamsAs1DForOutWhenUnconnected=off
  VarCompRatioPosCmd : Outport  Port=10  VectorParamsAs1DForOutWhenUnconnected=off
  IntkVlvLiftCmd : Outport  Port=11  VectorParamsAs1DForOutWhenUnconnected=off
  VarIntkRunLenCmd : Outport  Port=12  VectorParamsAs1DForOutWhenUnconnected=off
  ClsdLpFuelMult : Outport  Port=13  VectorParamsAs1DForOutWhenUnconnected=off
  IntkSwirlVlvPosCmd : Outport  Port=14  VectorParamsAs1DForOutWhenUnconnected=off
  TrqCmdISC : Outport  Port=15  VectorParamsAs1DForOutWhenUnconnected=off
  LoadCmd : Outport  Port=16  VectorParamsAs1DForOutWhenUnconnected=off
  EstIntkPortFlw : Outport  Port=17  VectorParamsAs1DForOutWhenUnconnected=off
  EngTrqCmd : Outport  Port=18  VectorParamsAs1DForOutWhenUnconnected=off
  StartCmd : Outport  Port=19  VectorParamsAs1DForOutWhenUnconnected=off
  MotTrqCmd : Outport  Port=20  VectorParamsAs1DForOutWhenUnconnected=off
  BrkCmd : Outport  Port=21  VectorParamsAs1DForOutWhenUnconnected=off
  GearCmd : Outport  Port=22  VectorParamsAs1DForOutWhenUnconnected=off
  Cltch1Cmd : Outport  Port=23  VectorParamsAs1DForOutWhenUnconnected=off
  wires:
  VarCompRatioPos/1 -> SiEngineController/11
  IntkVlvLift/1 -> SiEngineController/12
  VarIntkRunLen/1 -> SiEngineController/13
  Afr/1 -> SiEngineController/14
  IntkSwirlVlvPos/1 -> SiEngineController/15
  WgAreaPct/1 -> SiEngineController/6
  ThrPosPct/1 -> SiEngineController/5
  EgrVlvAreaPct/1 -> SiEngineController/10
  TurboRackPos/1 -> SiEngineController/9
  Mat/1 -> SiEngineController/4
  Map/1 -> SiEngineController/3
  EngSpd/1 -> SiEngineController/2
  TrqCmd/1 -> SiEngineController/1
  AmbPrs/1 -> SiEngineController/17
  TurboSpd/1 -> SiEngineController/16
  ExhCamPhase/1 -> SiEngineController/8
  IntkCamPhase/1 -> SiEngineController/7
  IgnSwtch/1 -> SiEngineController/18
  Hybrid Control Module (HCM)/1(EngTrqCmd) -> EngTrqCmd/1
  Hybrid Control Module (HCM)/5(StartCmd) -> StartCmd/1
  Hybrid Control Module (HCM)/3(BrkCmd) -> BrkCmd/1
  DecelPdl/1 -> Hybrid Control Module (HCM)/2(DecelPdl)
  EngSpdFdbk/1 -> Hybrid Control Module (HCM)/4(EngSpdFdbk)
  BattPwr/1 -> Hybrid Control Module (HCM)/6(BattPwr)
  BattSoc/1 -> Hybrid Control Module (HCM)/5(BattSoc)
  MotSpd/1 -> Hybrid Control Module (HCM)/7(MtrSpd)
  SiEngineController/1 -> ThrPosPctCmd/1
  SiEngineController/2 -> WgAreaPctCmd/1
  SiEngineController/3 -> InjPw/1
  SiEngineController/4 -> FuelMainSoi/1
  SiEngineController/5 -> SpdAdv/1
  SiEngineController/6 -> IntkCamPhaseCmd/1
  SiEngineController/7 -> ExhCamPhaseCmd/1
  SiEngineController/8 -> TurboRackPosCmd/1
  SiEngineController/9 -> EgrVlvAreaPctCmd/1
  SiEngineController/10 -> VarCompRatioPosCmd/1
  SiEngineController/11 -> IntkVlvLiftCmd/1
  SiEngineController/12 -> VarIntkRunLenCmd/1
  SiEngineController/13 -> ClsdLpFuelMult/1
  SiEngineController/14 -> IntkSwirlVlvPosCmd/1
  SiEngineController/15 -> TrqCmdISC/1
  SiEngineController/16 -> LoadCmd/1
  SiEngineController/17 -> EstIntkPortFlw/1
  Iat/1 -> SiEngineController/19
  Ect/1 -> SiEngineController/20
  EgrVlvDeltaPrs/1 -> SiEngineController/21
  EgrVlvInTemp/1 -> SiEngineController/22
  EngTrqOut/1 -> Hybrid Control Module (HCM)/8(EngTrqOut)
  Cltch2State/1 -> Hybrid Control Module (HCM)/10(Cltch2State)
  Cltch1State/1 -> Hybrid Control Module (HCM)/9(Cltch1State)
  AccelPdl/1 -> Hybrid Control Module (HCM)/1(AccelPdl), Transmission Control Module (TCM)/2
  VehSpdFdbk/1 -> Hybrid Control Module (HCM)/3(VehSpdFdbk), Transmission Control Module (TCM)/1
  Transmission Control Module (TCM)/1 -> GearCmd/1  "GearCmd"
  Hybrid Control Module (HCM)/6(Neutral) -> Transmission Control Module (TCM)/3
  Hybrid Control Module (HCM)/4(Cltch1Cmd) -> Cltch1Cmd/1
  Chrg/1 -> Hybrid Control Module (HCM)/11(Chrg)
  Hybrid Control Module (HCM)/2(MtrTrqCmd) -> MotTrqCmd/1
  BattV/1 -> Hybrid Control Module (HCM)/12(BattVolt)
  TransGear/1 -> Hybrid Control Module (HCM)/13(TransGear)
  Hybrid Control Module (HCM)/7(WhlTrqCmd) -> Terminator/1

== system HevP2ReferenceApplication/Longitudinal Driver/Longitudinal Driver ==
  Env : Inport
  Vref : Inport  Port=2
  Vfdbk : Inport  Port=3
  Bus Creator1 : BusCreator  Inputs=4
  Bus Selector : BusSelector  OutputSignals=Veh.xdot
  Bus Selector1 : BusSelector  OutputSignals=ErrMax
  Bus Selector2 : BusSelector  OutputSignals=Ground.Grade
  Constant : Constant  Value=false
  Data Type Conversion : DataTypeConversion  OutDataTypeStr=boolean  SaturateOnIntegerOverflow=off  RndMeth=Floor
  Hill Hold : Subsystem
  Ignition Switch Profile : Subsystem  Tag=STV Subsys  LoadFcn=sigbuilder_block('load');  StartFcn=sigbuilder_block('start');  StopFcn=sigbuilder_block('stop');  ClipboardFcn=sigbuilder_block('clipboard');  mask(Sigbuilder block){tuvar=[0:10]}
      mask help: Simulink:masks:SigbuilderBlock_MD
      mask init:
      | if ~strcmp(get_param(bdroot(gcbh),'SimulationStatus'),'stopped') tuvar = sigbuilder_block('maskInit'); end
      settings: CopyFcn=sigbuilder_block('copy');  DeleteFcn=sigbuilder_block('delete');  ModelCloseFcn=sigbuilder_block('modelClose');  PreSaveFcn=sigbuilder_block('preSave');  PauseFcn=sigbuilder_block('pause');  ContinueFcn=sigbuilder_block('continue');  NameChangeFcn=sigbuilder_block('namechange');  OpenFcn=sigbuilder_block('open',[595.8 176.4 550.8 322.2 ]);  CloseFcn=sigbuilder_block('close');
      mask Display: plot(0, 0, 100, 100,[2, 2, 32, 32, 2], [68, 8, 8, 68, 68],[32, 2], [38, 38], [32, 19, 2],[53, 60, 44], [32, 17, 17, 2],[16, 16, 31, 31]);txt = getActiveGroup(gcbh);text(2, 100, txt,'verticalAlignment', 'top');
  Longitudinal Driver Model : autolibshared/Longitudinal Driver  extAccelOvr=off  extDecelOvr=on  extAccelHld=off  extDecelHld=off  extAccelZero=on  extDecelZero=off  cntrlType=Predictive  shftType=Reverse, Neutral, Drive  velUnits=m/s  gearOut=off  Kp=1  Ki=1  Kff=0  Kg=0  VehVelVec=[0 100]  KffVec=[.1 .1]  KpVec=[10 10]  KiVec=[5 5]  KgVec=[0 0]  m=1623  Kpt=16337*2  tau=0.12  L=7  aR=159.22  bR=1.01  cR=0.3618  g=9.81  vnom=1  Kaw=0  tauerr=0  tauPt=2  GearInit=0  tShift=.1  pdlVec=[0.1 0.4 0.5 0.9]  upShftTbl=[-1 12.9375 26.4375 39.9375 51.18749999999999 62.4375 72.84375 83.25;-1 16.3125 29.8125 43.3125 54.5624 65.8125 76.78125 87.75;-1 19.6875 33.1875 46.68749999999999 57.9375 69.1875 80.71875 92.25;-1 33 52.5 77.25 100.5 138.75 161.875 185]  dwnShftTbl=[1 9.5625 23.0625 36.5625 47.8125 59.0625 68.90625 78.75;1 12.9375 26.4375 39.9375 51.18749999999999 62.4375 72.84375 83.25;1 16.3125 29.8125 43.3125 54.562499 65.8125 76.78125 87.75;1 19.6875 33.1875 46.68749999999999 57.9375 69.1875 80.71875 92.25]  tClutch=.5  tRev=.5  tPark=120  aMode=aMode  UpGearVec="[0  1  2  3  4  5  6  7]"  DownGearVec="[1  2  3  4  5  6  7  8]"
      settings: SourceProductBaseCode=PW,DR,MT,VE
  Manual Switch : ManualSwitch
  Optional Stationary Charging : Subsystem
  Terminator2 : Terminator
  OpCmds : Outport  VectorParamsAs1DForOutWhenUnconnected=off
  wires:
  Data Type Conversion/1 -> Manual Switch/2
  Longitudinal Driver Model/1 -> Bus Selector1/1  "Info"
  Longitudinal Driver Model/2 -> Bus Creator1/1  "Acc"
  Vref/1 -> Hill Hold/1(xdotref), Longitudinal Driver Model/1  "xdotref"
  Longitudinal Driver Model/3 -> Bus Creator1/2  "Dec"
  Vfdbk/1 -> Bus Selector/1, Hill Hold/2(VehFdbk)
  Manual Switch/1 -> Bus Creator1/3  "IgSw"
  Ignition Switch Profile/1(IGSW) -> Data Type Conversion/1
  Bus Selector/1 -> Longitudinal Driver Model/5  "<xdot>"
  Optional Stationary Charging/1(Charge) -> Bus Creator1/4  "Chrg"
  Bus Selector1/1 -> Terminator2/1  "<ErrMax>"
  Constant/1 -> Manual Switch/1
  Bus Creator1/1 -> OpCmds/1
  Bus Selector2/1 -> Hill Hold/3(Grade), Longitudinal Driver Model/6  "<Grade>"
  Hill Hold/1(EnblDecelOvr) -> Longitudinal Driver Model/2, Longitudinal Driver Model/3
  Hill Hold/2(DecelOvrCmd) -> Longitudinal Driver Model/4
  Env/1 -> Bus Selector2/1  "xdotref"

== system HevP2ReferenceApplication/Longitudinal Driver/Open Loop ==
  note: This subsystem is provided to disable the driver subsystem and expose the driver interface.
      |
      | The interface can:
      | - be connected with dashboard UI blocks or 3rd party hardware
      | - provide application specific pre-programmed event or time based signals
      | - be driven by recorded operator signals for tuning, troubleshooting and model validation
  Bus Creator1 : BusCreator  Inputs=4
  Constant : Constant  Value=false
  Constant1 : Constant  Value=0
  Constant2 : Constant  Value=0
  Data Type Conversion : DataTypeConversion  OutDataTypeStr=boolean  SaturateOnIntegerOverflow=off  RndMeth=Floor
  Ignition Switch Profile : Subsystem  Tag=STV Subsys  LoadFcn=sigbuilder_block('load');  StartFcn=sigbuilder_block('start');  StopFcn=sigbuilder_block('stop');  ClipboardFcn=sigbuilder_block('clipboard');  mask(Sigbuilder block){tuvar=[0:10]}
      mask help: Simulink:masks:SigbuilderBlock_MD
      mask init:
      | if ~strcmp(get_param(bdroot(gcbh),'SimulationStatus'),'stopped') tuvar = sigbuilder_block('maskInit'); end
      settings: CopyFcn=sigbuilder_block('copy');  DeleteFcn=sigbuilder_block('delete');  ModelCloseFcn=sigbuilder_block('modelClose');  PreSaveFcn=sigbuilder_block('preSave');  PauseFcn=sigbuilder_block('pause');  ContinueFcn=sigbuilder_block('continue');  NameChangeFcn=sigbuilder_block('namechange');  OpenFcn=sigbuilder_block('open',[595.8 176.4 550.8 322.2 ]);  CloseFcn=sigbuilder_block('close');
      mask Display: plot(0, 0, 100, 100,[2, 2, 32, 32, 2], [68, 8, 8, 68, 68],[32, 2], [38, 38], [32, 19, 2],[53, 60, 44], [32, 17, 17, 2],[16, 16, 31, 31]);txt = getActiveGroup(gcbh);text(2, 100, txt,'verticalAlignment', 'top');
  Manual Switch : ManualSwitch
  Optional Stationary Charging : Subsystem
  OpCmds : Outport  VectorParamsAs1DForOutWhenUnconnected=off
  wires:
  Bus Creator1/1 -> OpCmds/1
  Constant1/1 -> Bus Creator1/1  "Acc"
  Constant2/1 -> Bus Creator1/2  "Dec"
  Optional Stationary Charging/1(Charge) -> Bus Creator1/4  "Chrg"
  Ignition Switch Profile/1(IGSW) -> Data Type Conversion/1
  Constant/1 -> Manual Switch/1
  Manual Switch/1 -> Bus Creator1/3  "IgSw"
  Data Type Conversion/1 -> Manual Switch/2

== system HevP2ReferenceApplication/Passenger Car/Drivetrain ==
  note: 1) Add Subsystem or Model blocks as valid variant choices.
      | 2) You cannot connect blocks at this level. At simulation, connectivity is automatically
      | determined, based on the active variant and port name matching.
  Cltch1Cmd : Inport
  EngTrq : Inport  Port=2
  MotTrq : Inport  Port=3
  Grade : Inport  Port=4
  WindVel : Inport  Port=5
  BrkCmd : Inport  Port=6
  GearCmd : Inport  Port=7
  StartTrq : Inport  Port=8
  Drivetrain ptbs : ModelReference  ModelNameDialog=DrivetrainHevP2.slx  SimulationMode=Normal  VariantControl=Powertrain Blockset  ModelReferenceVersion=4.0
  Drivetrain ssc : ModelReference  ModelNameDialog=DrivetrainHevP2_SSC.slx  SimulationMode=Normal  VariantControl=Simscape  ModelReferenceVersion=4.24
  VehSpd : Outport  VectorParamsAs1DForOutWhenUnconnected=off
  EngSpd : Outport  Port=2  VectorParamsAs1DForOutWhenUnconnected=off  BusOutputAsStruct=on
  Cltch1State : Outport  Port=3  VectorParamsAs1DForOutWhenUnconnected=off  BusOutputAsStruct=on
  Cltch2State : Outport  Port=4  VectorParamsAs1DForOutWhenUnconnected=off  BusOutputAsStruct=on
  MotSpd : Outport  Port=5  VectorParamsAs1DForOutWhenUnconnected=off  BusOutputAsStruct=on
  TransGear : Outport  Port=6  VectorParamsAs1DForOutWhenUnconnected=off  BusOutputAsStruct=on

== system HevP2ReferenceApplication/Passenger Car/Drivetrain Output ==
  VehSpd : Inport
  "EngSpd " : Inport  Port=2
  Cltch1State : Inport  Port=3
  Cltch2State : Inport  Port=4
  MotSpd : Inport  Port=5
  TransGear : Inport  Port=6
  Bus Creator1 : BusCreator  Inputs=5
  Bus Creator3 : BusCreator  Inputs=1
  Sensor Dynamics : TransferFcn  Denominator=[0.01 1]
  VehFdbk : Outport  VectorParamsAs1DForOutWhenUnconnected=off
  EngFdbk : Outport  Port=2  VectorParamsAs1DForOutWhenUnconnected=off
  wires:
  "EngSpd "/1 -> Sensor Dynamics/1  "EngSpd"
  VehSpd/1 -> Bus Creator1/1  "xdot"
  TransGear/1 -> Bus Creator1/5  "TransGear"
  Cltch2State/1 -> Bus Creator1/3  "Cltch2State"
  MotSpd/1 -> Bus Creator1/4  "MotSpd"
  Cltch1State/1 -> Bus Creator1/2  "Cltch1State"
  Bus Creator3/1 -> EngFdbk/1  "EngFdbk"
  Sensor Dynamics/1 -> Bus Creator3/1  "EngSpd"
  Bus Creator1/1 -> VehFdbk/1  "VehFdbk"

== system HevP2ReferenceApplication/Passenger Car/Drivetrain Plant Input ==
  Ctrl : Inport
  EngFdbk : Inport  Port=2
  ElecFdbk : Inport  Port=3
  Env : Inport  Port=4
  Bus Selector : BusSelector  OutputSignals=PtCtrl.Cltch1Cmd,PtCtrl.BrkCmd,PtCtrl.GearCmd
  Bus Selector1 : BusSelector  OutputSignals=MotTrq,StartTrq
  Bus Selector2 : BusSelector  OutputSignals=EngTrq
  Bus Selector3 : BusSelector  OutputSignals=Ground.Grade,Wind.wind_x
  Engine Flex Plate Dynamics : TransferFcn  Denominator=[0.05 1]
  First Order Hold : FirstOrderHold  OutputAlgorithm=Fast (Minimize Error)  ErrorTolerance=10e6
  First Order Hold1 : FirstOrderHold  ErrorTolerance=10e6
  Rate Transition7 : RateTransition  Deterministic=off
  Cltch1Cmd : Outport  VectorParamsAs1DForOutWhenUnconnected=off
  EngTrq : Outport  Port=2  VectorParamsAs1DForOutWhenUnconnected=off
  MotTrq : Outport  Port=3  VectorParamsAs1DForOutWhenUnconnected=off
  Grade : Outport  Port=4  VectorParamsAs1DForOutWhenUnconnected=off
  WindVel : Outport  Port=5  VectorParamsAs1DForOutWhenUnconnected=off
  BrkCmd : Outport  Port=6  VectorParamsAs1DForOutWhenUnconnected=off
  GearCmd : Outport  Port=7  VectorParamsAs1DForOutWhenUnconnected=off
  StartTrq : Outport  Port=8  VectorParamsAs1DForOutWhenUnconnected=off
  wires:
  Bus Selector1/2 -> StartTrq/1  "<StartTrq>"
  Rate Transition7/1 -> GearCmd/1  "GearCmd"
  Bus Selector/3 -> Rate Transition7/1  "<GearCmd>"
  Bus Selector3/2 -> WindVel/1  "<wind_x>"
  Bus Selector3/1 -> Grade/1  "<Grade>"
  Env/1 -> Bus Selector3/1
  Bus Selector1/1 -> MotTrq/1  "<MotTrq>"
  ElecFdbk/1 -> Bus Selector1/1
  First Order Hold1/1 -> BrkCmd/1  "BrkCmd"
  First Order Hold/1 -> Cltch1Cmd/1  "Cltch1Cmd"
  Bus Selector/1 -> First Order Hold/1  "<Cltch1Cmd>"
  Bus Selector/2 -> First Order Hold1/1  "<BrkCmd>"
  EngFdbk/1 -> Bus Selector2/1
  Ctrl/1 -> Bus Selector/1
  Bus Selector2/1 -> Engine Flex Plate Dynamics/1  "<EngTrq>"
  Engine Flex Plate Dynamics/1 -> EngTrq/1  "EngineTrq"
